simulink model "LQR Based Yaw Moment Control Simulink"  (R2024b)
settings: Solver=FixedStepAuto  StartTime=0.0  StopTime=10  FixedStep=0.01  RelTol=1e-3
undefined symbols (not defined in the file): A, B, denominator, numerator
settings Model: Creator=Asus  LastModifiedBy=Asus
settings DataIOCC: ReturnWorkspaceOutputs=off

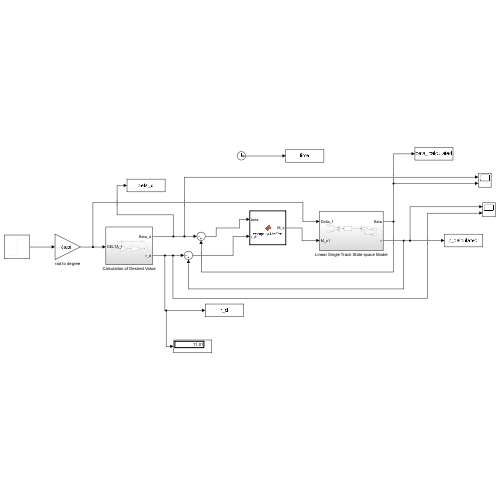
[thumbnail: Simulink's stored preview of the top-level diagram]
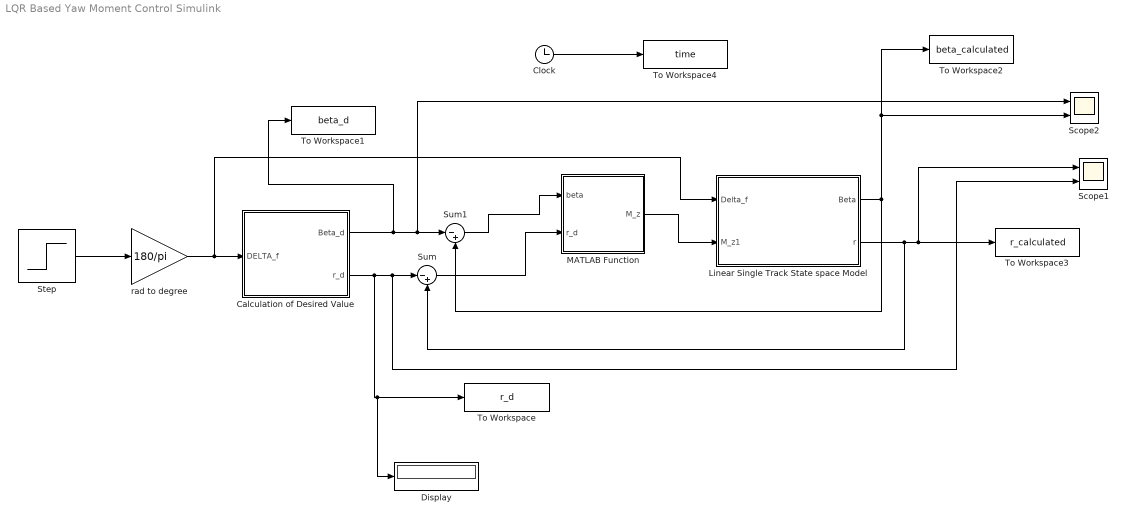
== system LQR Based Yaw Moment Control Simulink ==
  Calculation of Desired Value : Subsystem
  Clock : Clock
  Display : Display
  Linear Single Track State space Model : Subsystem
  MATLAB Function : MATLAB Function  TreatAsAtomicUnit=on
  Scope1 : Scope  NumInputPorts=2
  Scope2 : Scope  NumInputPorts=2
  Step : Step  After=2*pi/180  SampleTime=0
  Sum : Sum  Inputs=|-+
  Sum1 : Sum  Inputs=|-+
  To Workspace : ToWorkspace  VariableName=r_d  SampleTime=-1
      settings: Save2DSignal=2-D array (concatenate along first dimension)
  To Workspace1 : ToWorkspace  VariableName=beta_d  SampleTime=-1
      settings: Save2DSignal=2-D array (concatenate along first dimension)
  To Workspace2 : ToWorkspace  VariableName=beta_calculated  SampleTime=-1
      settings: Save2DSignal=2-D array (concatenate along first dimension)
  To Workspace3 : ToWorkspace  VariableName=r_calculated  SampleTime=-1
      settings: Save2DSignal=2-D array (concatenate along first dimension)
  To Workspace4 : ToWorkspace  VariableName=time  SampleTime=-1
      settings: Save2DSignal=2-D array (concatenate along first dimension)
  rad to degree : Gain  Gain=180/pi
  wires:
  Linear Single Track State space Model/1(Beta) -> Scope2/2, To Workspace2/1, Sum1/2
  Linear Single Track State space Model/2(r) -> Scope1/1, To Workspace3/1, Sum/2
  Calculation of Desired Value/2(r_d) -> Display/1, To Workspace/1, Scope1/2, Sum/1
  Calculation of Desired Value/1(Beta_d) -> To Workspace1/1, Scope2/1, Sum1/1
  Clock/1 -> To Workspace4/1
  Step/1 -> rad to degree/1
  Sum1/1 -> MATLAB Function/1(beta)
  Sum/1 -> MATLAB Function/2(r_d)
  MATLAB Function/1(M_z) -> Linear Single Track State space Model/2(M_z1)
  rad to degree/1 -> Linear Single Track State space Model/1(Delta_f), Calculation of Desired Value/1(DELTA_f)

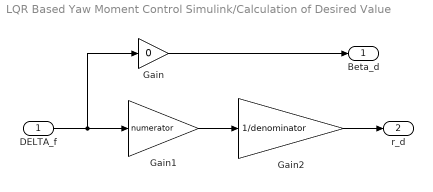
== system LQR Based Yaw Moment Control Simulink/Calculation of Desired Value ==
  DELTA_f : Inport
  Gain : Gain  Gain=0
  Gain1 : Gain  Gain=numerator
  Gain2 : Gain  Gain=1/denominator
  Beta_d : Outport
  r_d : Outport  Port=2
  wires:
  DELTA_f/1 -> Gain/1, Gain1/1
  Gain/1 -> Beta_d/1
  Gain1/1 -> Gain2/1
  Gain2/1 -> r_d/1

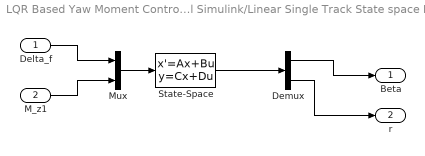
== system LQR Based Yaw Moment Control Simulink/Linear Single Track State space Model ==
  Delta_f : Inport
  M_z1 : Inport  Port=2
  Demux : Demux  Outputs=2
  Mux : Mux  Inputs=2
  State-Space : StateSpace  A=A  B=B  C=eye(2)  D=zeros(2)  InitialCondition=0
  Beta : Outport
  r : Outport  Port=2
  wires:
  Demux/1 -> Beta/1
  Demux/2 -> r/1
  State-Space/1 -> Demux/1
  Delta_f/1 -> Mux/1
  M_z1/1 -> Mux/2
  Mux/1 -> State-Space/1

== matlab function LQR Based Yaw Moment Control Simulink/MATLAB Function ==
  data: beta input; M_z output; r_d input
function M_z = computeMzFcn(beta,r_d)
    
    K1 =5.4849e+04	;
    K2 =2.9583e+05	;
    M_z = (-K1 * beta) + (-K2 * r_d);
end
